simulink model "pendulum_noratiobias"  (R2020b)
settings: Solver=ode15s  StartTime=0.0  StopTime=10.0  MaxStep=0.01  RelTol=1e-5  EnableMultiTasking=on
values from neighbouring files (symbols this model uses):
  d1 = 0.5    [simu.m]    (also in simu_J1fix.m)
  d2 = 0.5    [simu.m]    (also in simu_J1fix.m)
  is_tm1 = 1    [simu.m]    (also in simu_J1fix.m)
  is_tm2 = 1    [simu.m]    (also in simu_J1fix.m)
  Izz2 = 2    [simu.m]    (also in simu_J1fix.m)
  J1 = 1    [simu.m]    (also in simu_J1fix.m)
  J2 = 1    [simu.m]    (also in simu_J1fix.m = 0.8)
  k1 = 100    [simu.m]    (also in simu_J1fix.m)
  k2 = 100    [simu.m]    (also in simu_J1fix.m = 80)
  L1 = 0.4    [simu.m]    (also in simu_J1fix.m)
  L2 = 0.2    [simu.m]    (also in simu_J1fix.m)
  Lc2 = L2/2    (= 0.1)    [simu.m]    (also in simu_J1fix.m)
  lf1 = 1    [simu.m]    (also in simu_J1fix.m = 0.1)
  m2 = 1    [simu.m]    (also in simu_J1fix.m)
undefined symbols (not defined in the file or in its folder): X, Y, Z
libraries: nesl_utility x21, sm_lib x20, fl_lib x6
settings Model: Creator=BearHsia  LastModifiedBy=BearHsia
settings DataIOCC: LimitDataPoints=on  MaxDataPoints=10000
settings OptimizationCC: LifeSpan=inf
settings DebuggingCC: AllowSymbolicDim=off  SFUnexpectedBacktrackingDiag=warning  SFNoUnconditionalDefaultTransitionDiag=warning  SFExecutionAtInitializationDiag=none  ArithmeticOperatorsInVariantConditions=warning
settings SFSimCC: SimUseLocalCustomCode=off  CustomCodeUndefinedFunction=UseInterfaceOnly
settings RTWCC: RTWUseLocalCustomCode=off
settings CodeAppCC: StateflowObjectComments=on
settings GRTTargetCC: TargetLangStandard=C89/C90 (ANSI)
settings ConfigComp: CovMetricSettings=dw  CovSaveCumulativeToWorkspaceVar=on  CovSaveSingleToWorkspaceVar=on  CovExternalEMLEnable=off  CovSFcnEnable=off
settings SimscapeCC: SimscapeLogType=all  SimscapeLogSimulationStatistics=on  SimscapeLogDataHistory=10000

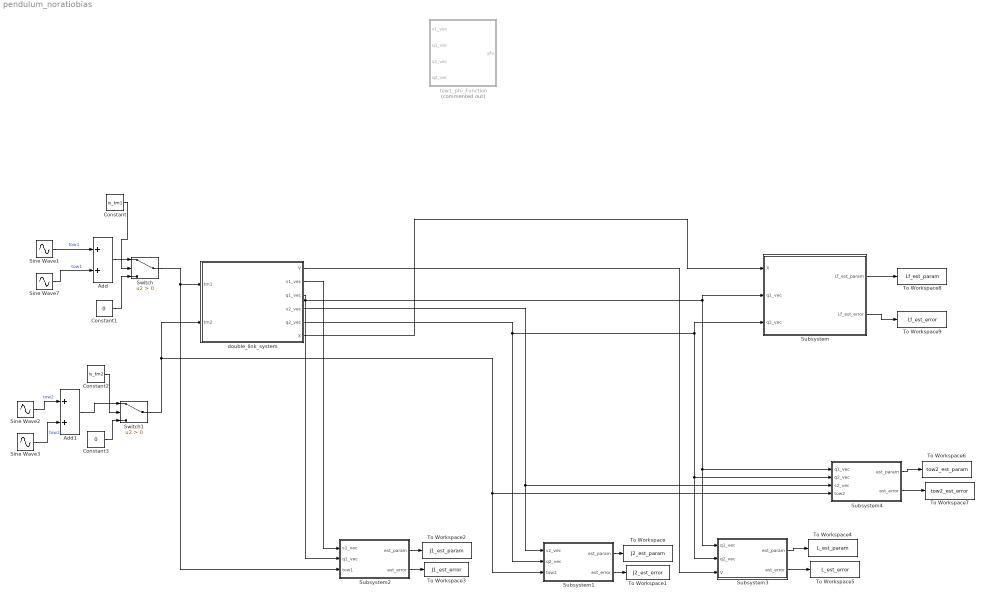
== system pendulum_noratiobias ==
  Add : Sum
  Add1 : Sum
  Constant : Constant  Value=is_tm1
  Constant1 : Constant  Value=0
  Constant2 : Constant  Value=is_tm2
  Constant3 : Constant  Value=0
  Sine Wave1 : Sin  Amplitude=2  SampleTime=0
  Sine Wave2 : Sin  Amplitude=2  SampleTime=0
  Sine Wave3 : Sin  Frequency=0.5  SampleTime=0
  Sine Wave7 : Sin  Frequency=0.5  SampleTime=0
  Subsystem : Subsystem
  Subsystem1 : Subsystem
  Subsystem2 : Subsystem
  Subsystem3 : Subsystem
  Subsystem4 : Subsystem
  Switch : Switch  Criteria=u2 > Threshold
  Switch1 : Switch  Criteria=u2 > Threshold
  To Workspace : ToWorkspace  VariableName=J2_est_param  SaveFormat=Timeseries  SampleTime=-1
  To Workspace1 : ToWorkspace  VariableName=J2_est_error  SaveFormat=Timeseries  SampleTime=-1
  To Workspace2 : ToWorkspace  VariableName=J1_est_param  SaveFormat=Timeseries  SampleTime=-1
  To Workspace3 : ToWorkspace  VariableName=J1_est_error  SaveFormat=Timeseries  SampleTime=-1
  To Workspace4 : ToWorkspace  VariableName=L_est_param  SaveFormat=Timeseries  SampleTime=-1
  To Workspace5 : ToWorkspace  VariableName=L_est_error  SaveFormat=Timeseries  SampleTime=-1
  To Workspace6 : ToWorkspace  VariableName=tow2_est_param  SaveFormat=Timeseries  SampleTime=-1
  To Workspace7 : ToWorkspace  VariableName=tow2_est_error  SaveFormat=Timeseries  SampleTime=-1
  To Workspace8 : ToWorkspace  VariableName=Lf_est_param  SaveFormat=Timeseries  SampleTime=-1
  To Workspace9 : ToWorkspace  VariableName=Lf_est_error  SaveFormat=Timeseries  SampleTime=-1
  double_link_system : Subsystem
  tow1_phi_Function : MATLAB Function  Commented=on  TreatAsAtomicUnit=on
  wires:
  double_link_system/2(s1_vec) -> Subsystem2/1(s1_vec)
  double_link_system/3(q1_vec) -> Subsystem/2(q1_vec), Subsystem4/1(q1_vec), Subsystem3/1(q1_vec), Subsystem2/2(q1_vec)
  Add/1 -> Switch/1
  Sine Wave1/1 -> Add/1  "tow1"
  Sine Wave7/1 -> Add/2  "tow1"
  double_link_system/4(s2_vec) -> Subsystem4/3(s2_vec), Subsystem1/1(s2_vec)
  double_link_system/5(q2_vec) -> Subsystem/3(q2_vec), Subsystem4/2(q2_vec), Subsystem3/2(q2_vec), Subsystem1/2(q2_vec)
  Subsystem1/1(est_param) -> To Workspace/1
  Subsystem1/2(est_error) -> To Workspace1/1
  Subsystem2/2(est_error) -> To Workspace3/1
  Subsystem2/1(est_param) -> To Workspace2/1
  Switch/1 -> Subsystem2/3(tow1), double_link_system/1(tm1)
  Constant/1 -> Switch/2
  Constant1/1 -> Switch/3
  Switch1/1 -> Subsystem4/4(tow2), Subsystem1/3(tow2), double_link_system/2(tm2)
  Constant2/1 -> Switch1/2
  Add1/1 -> Switch1/1
  Constant3/1 -> Switch1/3
  Sine Wave2/1 -> Add1/1  "tow2"
  Sine Wave3/1 -> Add1/2  "tow2"
  double_link_system/1(V) -> Subsystem3/3(V)
  Subsystem3/1(est_param) -> To Workspace4/1
  Subsystem3/2(est_error) -> To Workspace5/1
  Subsystem4/2(est_error) -> To Workspace7/1
  Subsystem4/1(est_param) -> To Workspace6/1
  double_link_system/6(X) -> Subsystem/1(X)
  Subsystem/1(Lf_est_param) -> To Workspace8/1
  Subsystem/2(Lf_est_error) -> To Workspace9/1

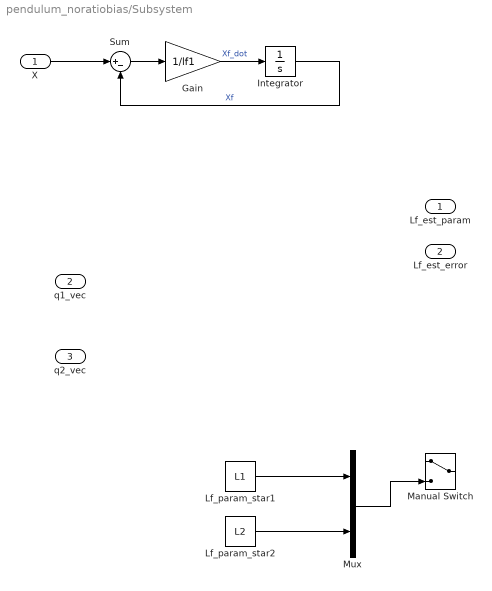
== system pendulum_noratiobias/Subsystem ==
  X : Inport
  q1_vec : Inport  Port=2
  q2_vec : Inport  Port=3
  Gain : Gain  Gain=1/lf1
  Integrator : Integrator
  Lf_param_star1 : Constant  Value=L1
  Lf_param_star2 : Constant  Value=L2
  Manual Switch : ManualSwitch
  Mux : Mux  Inputs=2
  Sum : Sum  Inputs=|+-
  Lf_est_param : Outport
  Lf_est_error : Outport  Port=2
  wires:
  Sum/1 -> Gain/1
  Gain/1 -> Integrator/1  "Xf_dot"
  X/1 -> Sum/1
  Integrator/1 -> Sum/2  "Xf"
  Mux/1 -> Manual Switch/2
  Lf_param_star1/1 -> Mux/1
  Lf_param_star2/1 -> Mux/2

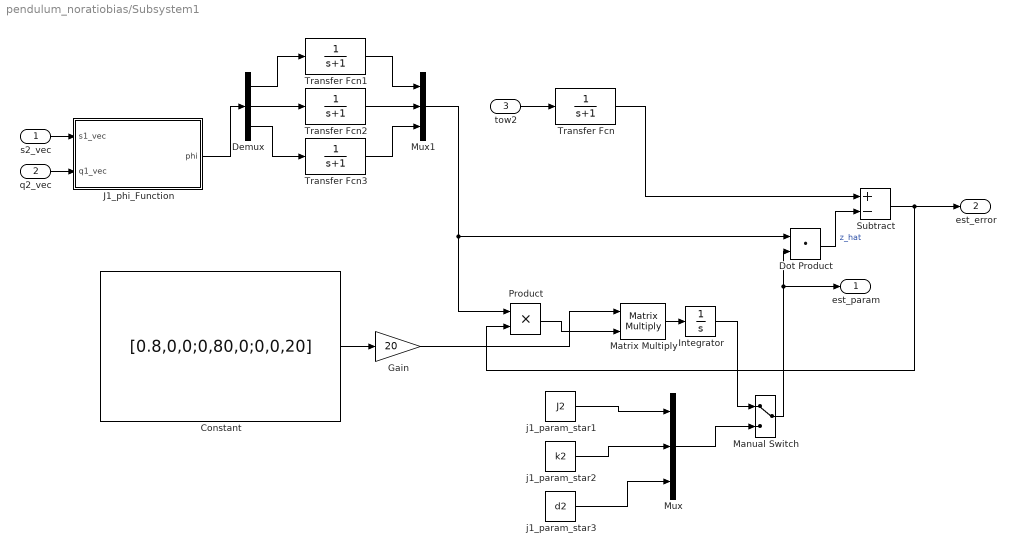
== system pendulum_noratiobias/Subsystem1 ==
  s2_vec : Inport
  q2_vec : Inport  Port=2
  tow2 : Inport  Port=3
  Constant : Constant  Value=[0.8,0,0;0,80,0;0,0,20]
  Demux : Demux  Outputs=3
  Dot Product : DotProduct  InputSameDT=on  OutDataTypeStr=Inherit: Inherit via internal rule
  Gain : Gain  Gain=20
  Integrator : Integrator  InitialCondition=[0.0001;0.0001;0.0001]
  J1_phi_Function : MATLAB Function  TreatAsAtomicUnit=on
  Manual Switch : ManualSwitch
  Matrix Multiply : Product  Multiplication=Matrix(*)
  Mux : Mux  Inputs=3
  Mux1 : Mux  Inputs=3
  Product : Product
  Subtract : Sum  Inputs=+-
  Transfer Fcn{,1..3} (4 alike) : TransferFcn  Denominator=[1 1]
  j1_param_star1 : Constant  Value=J2
  j1_param_star2 : Constant  Value=k2
  j1_param_star3 : Constant  Value=d2
  est_param : Outport
  est_error : Outport  Port=2
  wires:
  q2_vec/1 -> J1_phi_Function/2(q1_vec)
  s2_vec/1 -> J1_phi_Function/1(s1_vec)
  Integrator/1 -> Manual Switch/1
  tow2/1 -> Transfer Fcn/1
  Dot Product/1 -> Subtract/2  "z_hat"
  Matrix Multiply/1 -> Integrator/1
  Subtract/1 -> est_error/1, Product/2
  j1_param_star1/1 -> Mux/1
  j1_param_star2/1 -> Mux/2
  j1_param_star3/1 -> Mux/3
  Mux/1 -> Manual Switch/2
  Product/1 -> Matrix Multiply/2
  Gain/1 -> Matrix Multiply/1
  J1_phi_Function/1(phi) -> Demux/1
  Manual Switch/1 -> est_param/1, Dot Product/2
  Transfer Fcn/1 -> Subtract/1
  Transfer Fcn1/1 -> Mux1/1
  Transfer Fcn2/1 -> Mux1/2
  Transfer Fcn3/1 -> Mux1/3
  Demux/3 -> Transfer Fcn3/1
  Demux/2 -> Transfer Fcn2/1
  Demux/1 -> Transfer Fcn1/1
  Mux1/1 -> Product/1, Dot Product/1
  Constant/1 -> Gain/1

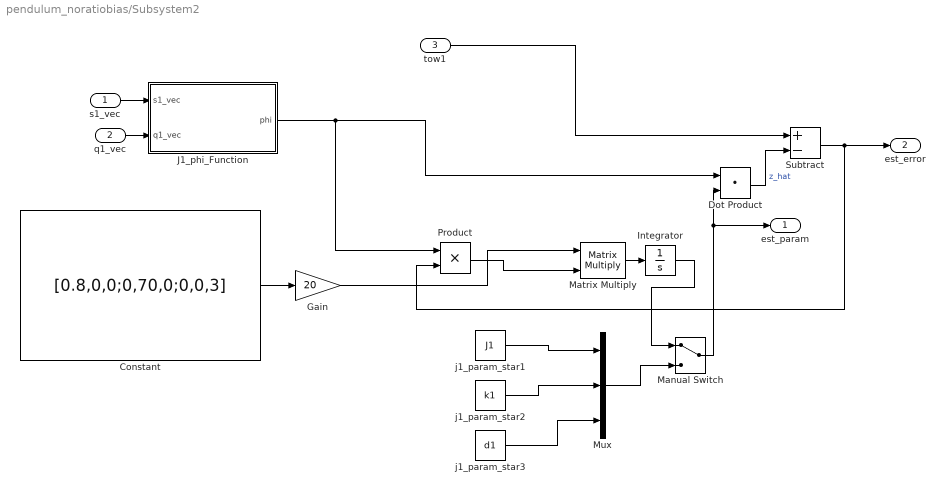
== system pendulum_noratiobias/Subsystem2 ==
  s1_vec : Inport
  q1_vec : Inport  Port=2
  tow1 : Inport  Port=3
  Constant : Constant  Value=[0.8,0,0;0,70,0;0,0,3]
  Dot Product : DotProduct  InputSameDT=on  OutDataTypeStr=Inherit: Inherit via internal rule
  Gain : Gain  Gain=20
  Integrator : Integrator  InitialCondition=[0;0;0]
  J1_phi_Function : MATLAB Function  TreatAsAtomicUnit=on
  Manual Switch : ManualSwitch
  Matrix Multiply : Product  Multiplication=Matrix(*)
  Mux : Mux  Inputs=3
  Product : Product
  Subtract : Sum  Inputs=+-
  j1_param_star1 : Constant  Value=J1
  j1_param_star2 : Constant  Value=k1
  j1_param_star3 : Constant  Value=d1
  est_param : Outport
  est_error : Outport  Port=2
  wires:
  q1_vec/1 -> J1_phi_Function/2(q1_vec)
  s1_vec/1 -> J1_phi_Function/1(s1_vec)
  Integrator/1 -> Manual Switch/1
  tow1/1 -> Subtract/1
  Dot Product/1 -> Subtract/2  "z_hat"
  Matrix Multiply/1 -> Integrator/1
  Subtract/1 -> est_error/1, Product/2
  j1_param_star1/1 -> Mux/1
  j1_param_star2/1 -> Mux/2
  j1_param_star3/1 -> Mux/3
  Mux/1 -> Manual Switch/2
  Product/1 -> Matrix Multiply/2
  Constant/1 -> Gain/1
  Gain/1 -> Matrix Multiply/1
  J1_phi_Function/1(phi) -> Dot Product/1, Product/1
  Manual Switch/1 -> est_param/1, Dot Product/2

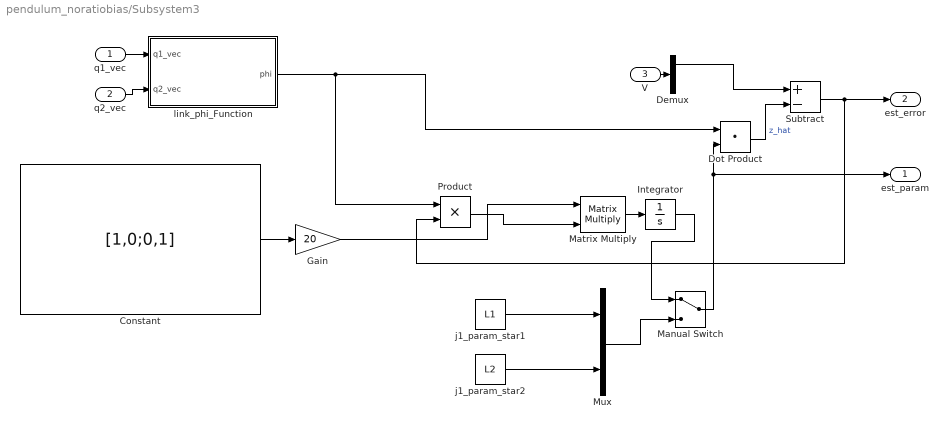
== system pendulum_noratiobias/Subsystem3 ==
  q1_vec : Inport
  q2_vec : Inport  Port=2
  V : Inport  Port=3
  Constant : Constant  Value=[1,0;0,1]
  Demux : Demux  Outputs=2
  Dot Product : DotProduct  InputSameDT=on  OutDataTypeStr=Inherit: Inherit via internal rule
  Gain : Gain  Gain=20
  Integrator : Integrator  InitialCondition=[0;0]
  Manual Switch : ManualSwitch
  Matrix Multiply : Product  Multiplication=Matrix(*)
  Mux : Mux  Inputs=2
  Product : Product
  Subtract : Sum  Inputs=+-
  j1_param_star1 : Constant  Value=L1
  j1_param_star2 : Constant  Value=L2
  link_phi_Function : MATLAB Function  TreatAsAtomicUnit=on
  est_param : Outport
  est_error : Outport  Port=2
  wires:
  Integrator/1 -> Manual Switch/1
  Dot Product/1 -> Subtract/2  "z_hat"
  Matrix Multiply/1 -> Integrator/1
  Subtract/1 -> est_error/1, Product/2
  j1_param_star1/1 -> Mux/1
  j1_param_star2/1 -> Mux/2
  Mux/1 -> Manual Switch/2
  Product/1 -> Matrix Multiply/2
  Constant/1 -> Gain/1
  Gain/1 -> Matrix Multiply/1
  link_phi_Function/1(phi) -> Dot Product/1, Product/1
  Manual Switch/1 -> est_param/1, Dot Product/2
  q2_vec/1 -> link_phi_Function/2(q2_vec)
  q1_vec/1 -> link_phi_Function/1(q1_vec)
  V/1 -> Demux/1
  Demux/1 -> Subtract/1

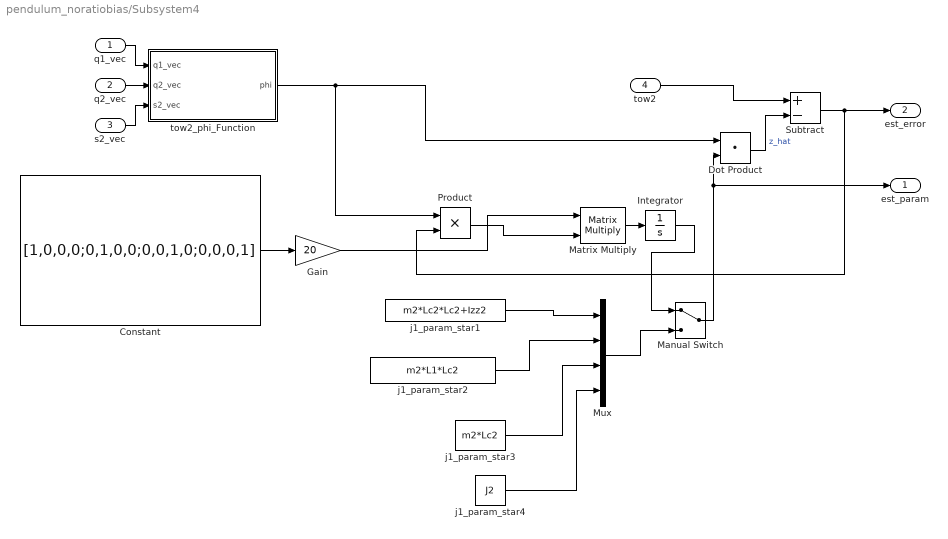
== system pendulum_noratiobias/Subsystem4 ==
  q1_vec : Inport
  q2_vec : Inport  Port=2
  s2_vec : Inport  Port=3
  tow2 : Inport  Port=4
  Constant : Constant  Value=[1,0,0,0;0,1,0,0;0,0,1,0;0,0,0,1]
  Dot Product : DotProduct  InputSameDT=on  OutDataTypeStr=Inherit: Inherit via internal rule
  Gain : Gain  Gain=20
  Integrator : Integrator  InitialCondition=[0;0;0;0]
  Manual Switch : ManualSwitch
  Matrix Multiply : Product  Multiplication=Matrix(*)
  Mux : Mux
  Product : Product
  Subtract : Sum  Inputs=+-
  j1_param_star1 : Constant  Value=m2*Lc2*Lc2+Izz2
  j1_param_star2 : Constant  Value=m2*L1*Lc2
  j1_param_star3 : Constant  Value=m2*Lc2
  j1_param_star4 : Constant  Value=J2
  tow2_phi_Function : MATLAB Function  TreatAsAtomicUnit=on
  est_param : Outport
  est_error : Outport  Port=2
  wires:
  Integrator/1 -> Manual Switch/1
  Dot Product/1 -> Subtract/2  "z_hat"
  Matrix Multiply/1 -> Integrator/1
  Subtract/1 -> est_error/1, Product/2
  j1_param_star1/1 -> Mux/1
  j1_param_star2/1 -> Mux/2
  Mux/1 -> Manual Switch/2
  Product/1 -> Matrix Multiply/2
  Constant/1 -> Gain/1
  Gain/1 -> Matrix Multiply/1
  tow2_phi_Function/1(phi) -> Dot Product/1, Product/1
  Manual Switch/1 -> est_param/1, Dot Product/2
  q2_vec/1 -> tow2_phi_Function/2(q2_vec)
  q1_vec/1 -> tow2_phi_Function/1(q1_vec)
  tow2/1 -> Subtract/1
  s2_vec/1 -> tow2_phi_Function/3(s2_vec)
  j1_param_star3/1 -> Mux/3
  j1_param_star4/1 -> Mux/4

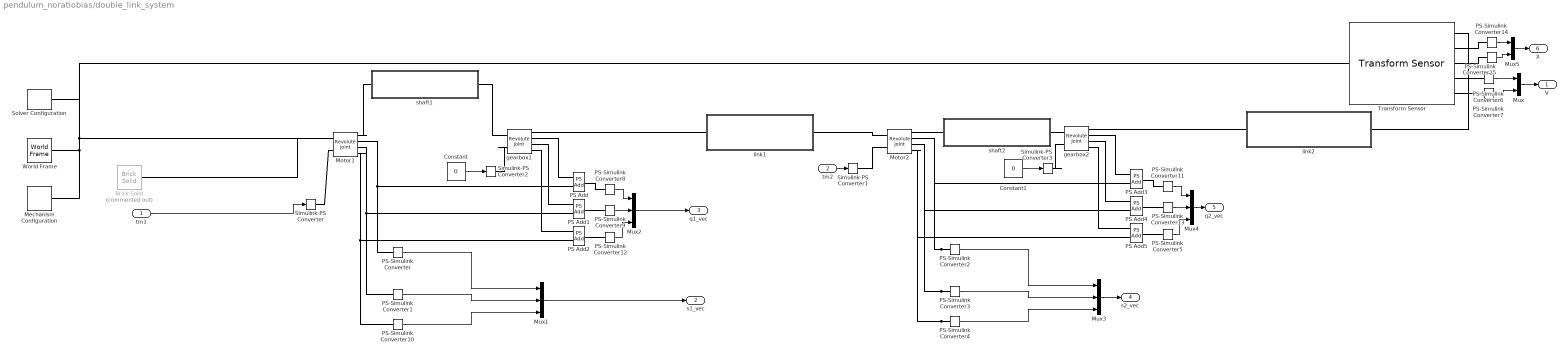
== system pendulum_noratiobias/double_link_system ==
  tm1 : Inport
  tm2 : Inport  Port=2
  Brick Solid : sm_lib/Body Elements/Brick Solid  Commented=on  GraphicAmbientColor=[0.15 0.15 0.15 1.0]  BasedOnType=Density  BrickDimensions=[4 4 4]  BrickDimensionUnits=cm  CenterOfMass=[0 0 0]  CenterOfMassUnits=m  GraphicDiffuseColor=[0.8 0.45 0]  Density=1000  DensityUnits=kg/m^3  DoExposeReferenceFrame=on  GraphicEmissiveColor=[0.0 0.0 0.0 1.0]  ExportEntireGeometry=off  SerializedFrames=<Frames/>  MarkerShape=Sphere  MarkerSize=10  GraphicType=FromGeometry  InertiaType=CalculateFromGeometry  Mass=1  MassUnits=kg  MomentsOfInertia=[1 1 1]  MomentsOfInertiaUnits=kg*m^2  GraphicOpacity=1.0  ProductsOfInertia=[0 0 0]  ProductsOfInertiaUnits=kg*m^2  GraphicShininess=75  GraphicSpecularColor=[0.5 0.5 0.5 1.0]  GraphicVisPropType=SimpleVisualProperties
  Constant : Constant  Value=0
  Constant1 : Constant  Value=0
  Mechanism Configuration : sm_lib/Utilities/Mechanism Configuration  UniformGravity=Constant  GravityVector=[0 -9.81 0]  GravityVectorUnits=m/s^2  GravityUnits=m/s^2  LinearizationDelta=0.001  JointModeTransitionNonlinearIterations=2
  Motor1 : sm_lib/Joints/Revolute Joint  JointMode=Normal  SenseConstraintForce=off  SenseConstraintForceX=off  SenseConstraintForceY=off  SenseConstraintForceZ=off  SenseConstraintTorque=off  SenseConstraintTorqueX=off  SenseConstraintTorqueY=off  SenseConstraintTorqueZ=off  SenseTotalForce=off  SenseTotalForceX=off  SenseTotalForceY=off  SenseTotalForceZ=off  SenseTotalTorque=off  SenseTotalTorqueX=off  SenseTotalTorqueY=off  SenseTotalTorqueZ=off  CompositeWrenchDir=FollowerOnBase  CompositeWrenchFrame=BaseFrame  EquilibriumPosition=-pi/2  EquilibriumPositionUnits=rad  SpringStiffness=0  SpringStiffnessUnits=N*m/rad  DampingCoefficient=0  DampingCoefficientUnits=N*m/(rad/s)  TorqueActuationMode=InputTorque  MotionActuationMode=ComputedMotion  SensePosition=on  SenseVelocity=on  SenseAcceleration=on  SenseTorqueForce=off  SenseLowerLimitTorqueForce=off  SenseUpperLimitTorqueForce=off  LowerLimitSpecify=off  LowerLimitBound=-90  LowerLimitBoundUnits=deg  LowerLimitStiffness=1e4  LowerLimitStiffnessUnits=N*m/deg  LowerLimitDamping=10  LowerLimitDampingUnits=N*m/(deg/s)  LowerLimitTransitionRegionWidth=0.1  LowerLimitTransitionRegionWidthUnits=deg  UpperLimitSpecify=off  UpperLimitBound=90  UpperLimitBoundUnits=deg  UpperLimitStiffness=1e4  UpperLimitStiffnessUnits=N*m/deg  UpperLimitDamping=10  UpperLimitDampingUnits=N*m/(deg/s)  UpperLimitTransitionRegionWidth=0.1  UpperLimitTransitionRegionWidthUnits=deg  PositionTargetSpecify=on  PositionTargetPriority=High  PositionTargetValue=-pi/2  PositionTargetValueUnits=rad  VelocityTargetSpecify=off  VelocityTargetPriority=High  VelocityTargetValue=0  VelocityTargetValueUnits=deg/s
  Motor2 : sm_lib/Joints/Revolute Joint  JointMode=Normal  SenseConstraintForce=off  SenseConstraintForceX=off  SenseConstraintForceY=off  SenseConstraintForceZ=off  SenseConstraintTorque=off  SenseConstraintTorqueX=off  SenseConstraintTorqueY=off  SenseConstraintTorqueZ=off  SenseTotalForce=off  SenseTotalForceX=off  SenseTotalForceY=off  SenseTotalForceZ=off  SenseTotalTorque=off  SenseTotalTorqueX=off  SenseTotalTorqueY=off  SenseTotalTorqueZ=off  CompositeWrenchDir=FollowerOnBase  CompositeWrenchFrame=BaseFrame  EquilibriumPosition=0  EquilibriumPositionUnits=rad  SpringStiffness=0  SpringStiffnessUnits=N*m/rad  DampingCoefficient=0  DampingCoefficientUnits=N*m/(rad/s)  TorqueActuationMode=InputTorque  MotionActuationMode=ComputedMotion  SensePosition=on  SenseVelocity=on  SenseAcceleration=on  SenseTorqueForce=off  SenseLowerLimitTorqueForce=off  SenseUpperLimitTorqueForce=off  LowerLimitSpecify=off  LowerLimitBound=-90  LowerLimitBoundUnits=deg  LowerLimitStiffness=1e4  LowerLimitStiffnessUnits=N*m/deg  LowerLimitDamping=10  LowerLimitDampingUnits=N*m/(deg/s)  LowerLimitTransitionRegionWidth=0.1  LowerLimitTransitionRegionWidthUnits=deg  UpperLimitSpecify=off  UpperLimitBound=90  UpperLimitBoundUnits=deg  UpperLimitStiffness=1e4  UpperLimitStiffnessUnits=N*m/deg  UpperLimitDamping=10  UpperLimitDampingUnits=N*m/(deg/s)  UpperLimitTransitionRegionWidth=0.1  UpperLimitTransitionRegionWidthUnits=deg  PositionTargetSpecify=on  PositionTargetPriority=High  PositionTargetValue=0  PositionTargetValueUnits=rad  VelocityTargetSpecify=off  VelocityTargetPriority=High  VelocityTargetValue=0  VelocityTargetValueUnits=deg/s
  Mux : Mux  Inputs=2
  Mux{1..4} (4 alike) : Mux  Inputs=3
  Mux5 : Mux  Inputs=2
  PS Add{,1..5} (6 alike) : fl_lib/Physical Signals/Functions/PS Add
  PS-Simulink Converter{,1..15} (16 alike) : nesl_utility/PS-Simulink Converter  PhysicalDomain=network_engine_domain  SubClassName=ps_output  LeftPortType=input  RightPortType=output  PseudoPeriodic=off  Frequencies=[]  Unit=inherit  AffineConversion=off
  Simulink-PS Converter{,1..3} (4 alike) : nesl_utility/Simulink-PS Converter  PhysicalDomain=network_engine_domain  SubClassName=ps_input  LeftPortType=input  RightPortType=output  PseudoPeriodic=off  Frequencies=[]  NoiseDistribution=none  NoiseParameters=[]  Unit=1  AffineConversion=off  FilteringAndDerivatives=provide  SimscapeFilterOrder=1  InputFilterTimeConstant=0.001  UdotUserProvided=0
  Solver Configuration : nesl_utility/Solver Configuration  PhysicalDomain=network_engine_domain  SubClassName=solver  LeftPortType=input  RightPortType=generic  Tones=[]  Harmonics=[]  SimulateNoise=off  Profile=off  UseLocalSampling=off  EnableSwitchedLinearOptims=on  FrequencyDomain=off  UseCCode=off  RelTol=0.001  AbsTol=1e-06  MinStep=1e-09  ToWorkspace=off  RevertToSquareIcSolve=off  NumHomotopyIterations=100  PhasorMode=off  PhasorModeNumHarmonics=1  DoDC=on  ResidualTolerance=1e-09  UseLocalSolver=off  LocalSolverChoice=NE_BACKWARD_EULER_ADVANCER  LocalSolverSampleTime=0.001  DoFixedCost=off  MaxNonlinIter=3  MaxModeIter=2  ComputeImpulses=off  ImpulseIterations=2  LinearAlgebra=Sparse  EquationFormulation=NE_TIME_EF  DelaysMemoryBudget=1024  AutomaticFiltering=on  FilteringTimeConstant=0.001  PartitionStorageMethod=AS_NEEDED  PartitionMemoryBudget=1024  PartitionMethod=FAST
  Transform Sensor : sm_lib/Frames and Transforms/Transform Sensor  MeasurementFrame=World  SenseAngle=off  SenseAxis=off  SenseAngle1=off  SenseAngle2=off  SenseAngle3=off  SenseQ=off  SenseR=off  SenseOmegaX=off  SenseOmegaY=off  SenseOmegaZ=off  SenseOmega1=off  SenseOmega2=off  SenseOmega3=off  SenseQDot=off  SenseRDot=off  SenseAlphaX=off  SenseAlphaY=off  SenseAlphaZ=off  SenseAlpha1=off  SenseAlpha2=off  SenseAlpha3=off  SenseQDDot=off  SenseRDDot=off  SenseX=on  SenseY=on  SenseZ=off  SenseRad=off  SenseAzim=off  SenseDist=off  SenseInc=off  SenseXDot=on  SenseYDot=on  SenseZDot=off  SenseRadDot=off  SenseAzimDot=off  SenseDistDot=off  SenseIncDot=off  SenseXDDot=off  SenseYDDot=off  SenseZDDot=off  SenseRadDDot=off  SenseAzimDDot=off  SenseDistDDot=off  SenseIncDDot=off
  World Frame : sm_lib/Frames and Transforms/World Frame
  gearbox1 : sm_lib/Joints/Revolute Joint  JointMode=Normal  SenseConstraintForce=off  SenseConstraintForceX=off  SenseConstraintForceY=off  SenseConstraintForceZ=off  SenseConstraintTorque=off  SenseConstraintTorqueX=off  SenseConstraintTorqueY=off  SenseConstraintTorqueZ=off  SenseTotalForce=off  SenseTotalForceX=off  SenseTotalForceY=off  SenseTotalForceZ=off  SenseTotalTorque=off  SenseTotalTorqueX=off  SenseTotalTorqueY=off  SenseTotalTorqueZ=off  CompositeWrenchDir=FollowerOnBase  CompositeWrenchFrame=BaseFrame  EquilibriumPosition=0  EquilibriumPositionUnits=rad  SpringStiffness=k1  SpringStiffnessUnits=N*m/rad  DampingCoefficient=d1  DampingCoefficientUnits=N*m/(rad/s)  TorqueActuationMode=InputTorque  MotionActuationMode=ComputedMotion  SensePosition=on  SenseVelocity=on  SenseAcceleration=on  SenseTorqueForce=off  SenseLowerLimitTorqueForce=off  SenseUpperLimitTorqueForce=off  LowerLimitSpecify=off  LowerLimitBound=-90  LowerLimitBoundUnits=deg  LowerLimitStiffness=1e4  LowerLimitStiffnessUnits=N*m/deg  LowerLimitDamping=10  LowerLimitDampingUnits=N*m/(deg/s)  LowerLimitTransitionRegionWidth=0.1  LowerLimitTransitionRegionWidthUnits=deg  UpperLimitSpecify=off  UpperLimitBound=90  UpperLimitBoundUnits=deg  UpperLimitStiffness=1e4  UpperLimitStiffnessUnits=N*m/deg  UpperLimitDamping=10  UpperLimitDampingUnits=N*m/(deg/s)  UpperLimitTransitionRegionWidth=0.1  UpperLimitTransitionRegionWidthUnits=deg  PositionTargetSpecify=on  PositionTargetPriority=High  PositionTargetValue=0  PositionTargetValueUnits=rad  VelocityTargetSpecify=off  VelocityTargetPriority=High  VelocityTargetValue=0  VelocityTargetValueUnits=deg/s
  gearbox2 : sm_lib/Joints/Revolute Joint  JointMode=Normal  SenseConstraintForce=off  SenseConstraintForceX=off  SenseConstraintForceY=off  SenseConstraintForceZ=off  SenseConstraintTorque=off  SenseConstraintTorqueX=off  SenseConstraintTorqueY=off  SenseConstraintTorqueZ=off  SenseTotalForce=off  SenseTotalForceX=off  SenseTotalForceY=off  SenseTotalForceZ=off  SenseTotalTorque=off  SenseTotalTorqueX=off  SenseTotalTorqueY=off  SenseTotalTorqueZ=off  CompositeWrenchDir=FollowerOnBase  CompositeWrenchFrame=BaseFrame  EquilibriumPosition=0  EquilibriumPositionUnits=rad  SpringStiffness=k2  SpringStiffnessUnits=N*m/rad  DampingCoefficient=d2  DampingCoefficientUnits=N*m/(rad/s)  TorqueActuationMode=InputTorque  MotionActuationMode=ComputedMotion  SensePosition=on  SenseVelocity=on  SenseAcceleration=on  SenseTorqueForce=off  SenseLowerLimitTorqueForce=off  SenseUpperLimitTorqueForce=off  LowerLimitSpecify=off  LowerLimitBound=-90  LowerLimitBoundUnits=deg  LowerLimitStiffness=1e4  LowerLimitStiffnessUnits=N*m/deg  LowerLimitDamping=10  LowerLimitDampingUnits=N*m/(deg/s)  LowerLimitTransitionRegionWidth=0.1  LowerLimitTransitionRegionWidthUnits=deg  UpperLimitSpecify=off  UpperLimitBound=90  UpperLimitBoundUnits=deg  UpperLimitStiffness=1e4  UpperLimitStiffnessUnits=N*m/deg  UpperLimitDamping=10  UpperLimitDampingUnits=N*m/(deg/s)  UpperLimitTransitionRegionWidth=0.1  UpperLimitTransitionRegionWidthUnits=deg  PositionTargetSpecify=on  PositionTargetPriority=High  PositionTargetValue=0  PositionTargetValueUnits=rad  VelocityTargetSpecify=off  VelocityTargetPriority=High  VelocityTargetValue=0  VelocityTargetValueUnits=deg/s
  link1 : Subsystem  mask{rgb=[0.25 0.4 0.7], Ixx=1, Iyy=1, Izz=3, M=1, L=L1, W=0.04, H=0.04}
      mask prompts: rgb "Color [R G B]"
  link2 : Subsystem  mask{rgb=[0.25 0.4 0.7], Ixx=1, Iyy=1, Izz=Izz2, M=m2, L=L2, W=0.04, H=0.04}
      mask prompts: rgb "Color [R G B]"
  shaft1 : Subsystem  mask{rgb=[0 1 0], Ixx=0, Iyy=0, Izz=J1, M=0.1, L=0.2, W=0.004, H=0.004}
      mask prompts: rgb "Color [R G B]"
  shaft2 : Subsystem  mask{rgb=[0 1 0], Ixx=0, Iyy=0, Izz=J2, M=0.1, L=0.2, W=0.004, H=0.004}
      mask prompts: rgb "Color [R G B]"
  V : Outport
  s1_vec : Outport  Port=2
  q1_vec : Outport  Port=3
  s2_vec : Outport  Port=4
  q2_vec : Outport  Port=5
  X : Outport  Port=6
  wires:
  tm2/1 -> Simulink-PS Converter1/1
  tm1/1 -> Simulink-PS Converter/1
  PS-Simulink Converter6/1 -> Mux/1
  PS-Simulink Converter7/1 -> Mux/2
  Mux/1 -> V/1
  PS-Simulink Converter9/1 -> Mux2/2
  PS-Simulink Converter8/1 -> Mux2/1
  PS-Simulink Converter12/1 -> Mux2/3
  Mux1/1 -> s1_vec/1
  Mux2/1 -> q1_vec/1
  PS-Simulink Converter/1 -> Mux1/1
  PS-Simulink Converter1/1 -> Mux1/2
  PS-Simulink Converter10/1 -> Mux1/3
  Mux3/1 -> s2_vec/1
  PS-Simulink Converter2/1 -> Mux3/1
  PS-Simulink Converter4/1 -> Mux3/3
  PS-Simulink Converter5/1 -> Mux4/3
  PS-Simulink Converter11/1 -> Mux4/1
  Mux4/1 -> q2_vec/1
  PS-Simulink Converter13/1 -> Mux4/2
  PS-Simulink Converter3/1 -> Mux3/2
  Constant/1 -> Simulink-PS Converter2/1
  Constant1/1 -> Simulink-PS Converter3/1
  Mux5/1 -> X/1
  PS-Simulink Converter14/1 -> Mux5/1
  PS-Simulink Converter15/1 -> Mux5/2
  connections:
  Simulink-PS Converter/RConn1 -- Motor1/LConn2
  World Frame/RConn1 -- Mechanism Configuration/RConn1 -- Transform Sensor/LConn1 -- Solver Configuration/RConn1 -- Brick Solid/RConn1 -- Motor1/LConn1
  Motor1/RConn4 -- PS Add2/LConn2 -- PS-Simulink Converter10/LConn1
  Motor1/RConn2 -- PS Add/LConn2 -- PS-Simulink Converter/LConn1
  link2/RConn1 -- Transform Sensor/RConn1
  Transform Sensor/RConn5 -- PS-Simulink Converter7/LConn1
  gearbox1/RConn3 -- PS Add1/LConn1
  PS Add1/RConn1 -- PS-Simulink Converter9/LConn1
  gearbox1/RConn4 -- PS Add2/LConn1
  PS Add/RConn1 -- PS-Simulink Converter8/LConn1
  Motor1/RConn3 -- PS Add1/LConn2 -- PS-Simulink Converter1/LConn1
  Transform Sensor/RConn4 -- PS-Simulink Converter6/LConn1
  gearbox1/RConn2 -- PS Add/LConn1
  PS-Simulink Converter12/LConn1 -- PS Add2/RConn1
  PS-Simulink Converter4/LConn1 -- Motor2/RConn4 -- PS Add5/LConn2
  PS-Simulink Converter3/LConn1 -- Motor2/RConn3 -- PS Add4/LConn2
  PS-Simulink Converter2/LConn1 -- Motor2/RConn2 -- PS Add3/LConn2
  gearbox2/RConn1 -- link2/LConn1
  gearbox2/RConn2 -- PS Add3/LConn1
  shaft2/LConn1 -- Motor2/RConn1
  gearbox2/RConn3 -- PS Add4/LConn1
  PS-Simulink Converter5/LConn1 -- PS Add5/RConn1
  PS Add3/RConn1 -- PS-Simulink Converter11/LConn1
  shaft2/RConn1 -- gearbox2/LConn1
  gearbox2/RConn4 -- PS Add5/LConn1
  PS Add4/RConn1 -- PS-Simulink Converter13/LConn1
  link1/RConn1 -- Motor2/LConn1
  Simulink-PS Converter1/RConn1 -- Motor2/LConn2
  gearbox1/LConn2 -- Simulink-PS Converter2/RConn1
  Simulink-PS Converter3/RConn1 -- gearbox2/LConn2
  Motor1/RConn1 -- shaft1/LConn1
  shaft1/RConn1 -- gearbox1/LConn1
  gearbox1/RConn1 -- link1/LConn1
  Transform Sensor/RConn2 -- PS-Simulink Converter14/LConn1
  Transform Sensor/RConn3 -- PS-Simulink Converter15/LConn1

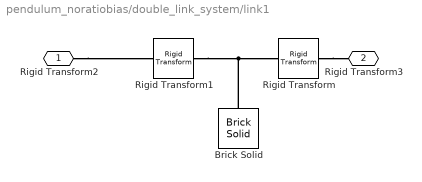
== system pendulum_noratiobias/double_link_system/link1 ==
  Brick Solid : sm_lib/Body Elements/Brick Solid  GraphicAmbientColor=[0.15 0.15 0.15 1.0]  BasedOnType=Density  BrickDimensions=[L W H]  BrickDimensionUnits=m  CenterOfMass=[0 0 0]  CenterOfMassUnits=m  GraphicDiffuseColor=rgb  Density=2700  DensityUnits=kg/m^3  DoExposeReferenceFrame=on  GraphicEmissiveColor=[0.0 0.0 0.0 1.0]  ExportEntireGeometry=off  SerializedFrames=<Frames/>  MarkerShape=Sphere  MarkerSize=10  GraphicType=FromGeometry  InertiaType=Custom  Mass=M  MassUnits=kg  MomentsOfInertia=[Ixx Iyy Izz]  MomentsOfInertiaUnits=kg*m^2  GraphicOpacity=1.0  ProductsOfInertia=[0 0 0]  ProductsOfInertiaUnits=kg*m^2  GraphicShininess=75  GraphicSpecularColor=[0.5 0.5 0.5 1.0]  GraphicVisPropType=SimpleVisualProperties
  Rigid Transform : sm_lib/Frames and Transforms/Rigid Transform  TranslationMethod=StandardAxis  TranslationStandardOffset=L/2  TranslationLengthUnit=m  TranslationStandardAxis=+X  TranslationCartesianOffset=[0 0 0]  TranslationROffset=0  TranslationROffsetUnits=m  TranslationZOffset=0  TranslationZOffsetUnits=m  TranslationThetaOffset=0  TranslationThetaOffsetUnits=deg  RotationMethod=None  RotationAngleUnits=deg  RotationStandardAxis=+Z  RotationAngle=0.0  RotationArbitraryAxis=[0 0 1]  FollAlignAxisA=+X  BaseAlignAxisA=+Y  FollAlignAxisB=+Y  BaseAlignAxisB=+Z  RotationSequenceAxes=FollowerAxes  RotationSequence=XYX  RotationSequenceAngles=[0 0 0]  RotationSequenceAnglesUnits=deg  RotationMatrix=[1 0 0; 0 1 0; 0 0 1]
  Rigid Transform1 : sm_lib/Frames and Transforms/Rigid Transform  TranslationMethod=StandardAxis  TranslationStandardOffset=L/2  TranslationLengthUnit=m  TranslationStandardAxis=-X  TranslationCartesianOffset=[0 0 0]  TranslationROffset=0  TranslationROffsetUnits=m  TranslationZOffset=0  TranslationZOffsetUnits=m  TranslationThetaOffset=0  TranslationThetaOffsetUnits=deg  RotationMethod=None  RotationAngleUnits=deg  RotationStandardAxis=-X  RotationAngle=0.0  RotationArbitraryAxis=[0 0 1]  FollAlignAxisA=+X  BaseAlignAxisA=+Y  FollAlignAxisB=+Y  BaseAlignAxisB=+Z  RotationSequenceAxes=FollowerAxes  RotationSequence=XYX  RotationSequenceAngles=[0 0 0]  RotationSequenceAnglesUnits=deg  RotationMatrix=[1 0 0; 0 1 0; 0 0 1]
  Rigid Transform2 : PMIOPort  Side=Left
  Rigid Transform3 : PMIOPort  Port=2  Side=Right
  connections:
  Rigid Transform1/LConn1 -- Rigid Transform/LConn1 -- Brick Solid/RConn1
  Rigid Transform/RConn1 -- Rigid Transform3/RConn1
  Rigid Transform2/RConn1 -- Rigid Transform1/RConn1

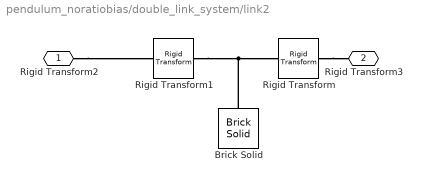
== system pendulum_noratiobias/double_link_system/link2 ==
  Brick Solid : sm_lib/Body Elements/Brick Solid  GraphicAmbientColor=[0.15 0.15 0.15 1.0]  BasedOnType=Density  BrickDimensions=[L W H]  BrickDimensionUnits=m  CenterOfMass=[0 0 0]  CenterOfMassUnits=m  GraphicDiffuseColor=rgb  Density=2700  DensityUnits=kg/m^3  DoExposeReferenceFrame=on  GraphicEmissiveColor=[0.0 0.0 0.0 1.0]  ExportEntireGeometry=off  SerializedFrames=<Frames/>  MarkerShape=Sphere  MarkerSize=10  GraphicType=FromGeometry  InertiaType=Custom  Mass=M  MassUnits=kg  MomentsOfInertia=[Ixx Iyy Izz]  MomentsOfInertiaUnits=kg*m^2  GraphicOpacity=1.0  ProductsOfInertia=[0 0 0]  ProductsOfInertiaUnits=kg*m^2  GraphicShininess=75  GraphicSpecularColor=[0.5 0.5 0.5 1.0]  GraphicVisPropType=SimpleVisualProperties
  Rigid Transform : sm_lib/Frames and Transforms/Rigid Transform  TranslationMethod=StandardAxis  TranslationStandardOffset=L/2  TranslationLengthUnit=m  TranslationStandardAxis=+X  TranslationCartesianOffset=[0 0 0]  TranslationROffset=0  TranslationROffsetUnits=m  TranslationZOffset=0  TranslationZOffsetUnits=m  TranslationThetaOffset=0  TranslationThetaOffsetUnits=deg  RotationMethod=None  RotationAngleUnits=deg  RotationStandardAxis=+Z  RotationAngle=0.0  RotationArbitraryAxis=[0 0 1]  FollAlignAxisA=+X  BaseAlignAxisA=+Y  FollAlignAxisB=+Y  BaseAlignAxisB=+Z  RotationSequenceAxes=FollowerAxes  RotationSequence=XYX  RotationSequenceAngles=[0 0 0]  RotationSequenceAnglesUnits=deg  RotationMatrix=[1 0 0; 0 1 0; 0 0 1]
  Rigid Transform1 : sm_lib/Frames and Transforms/Rigid Transform  TranslationMethod=StandardAxis  TranslationStandardOffset=L/2  TranslationLengthUnit=m  TranslationStandardAxis=-X  TranslationCartesianOffset=[0 0 0]  TranslationROffset=0  TranslationROffsetUnits=m  TranslationZOffset=0  TranslationZOffsetUnits=m  TranslationThetaOffset=0  TranslationThetaOffsetUnits=deg  RotationMethod=None  RotationAngleUnits=deg  RotationStandardAxis=-X  RotationAngle=0.0  RotationArbitraryAxis=[0 0 1]  FollAlignAxisA=+X  BaseAlignAxisA=+Y  FollAlignAxisB=+Y  BaseAlignAxisB=+Z  RotationSequenceAxes=FollowerAxes  RotationSequence=XYX  RotationSequenceAngles=[0 0 0]  RotationSequenceAnglesUnits=deg  RotationMatrix=[1 0 0; 0 1 0; 0 0 1]
  Rigid Transform2 : PMIOPort  Side=Left
  Rigid Transform3 : PMIOPort  Port=2  Side=Right
  connections:
  Rigid Transform1/LConn1 -- Rigid Transform/LConn1 -- Brick Solid/RConn1
  Rigid Transform/RConn1 -- Rigid Transform3/RConn1
  Rigid Transform2/RConn1 -- Rigid Transform1/RConn1

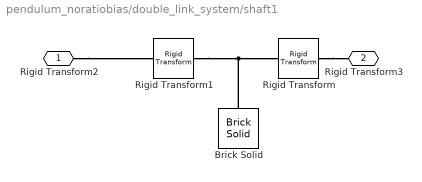
== system pendulum_noratiobias/double_link_system/shaft1 ==
  Brick Solid : sm_lib/Body Elements/Brick Solid  GraphicAmbientColor=[0.15 0.15 0.15 1.0]  BasedOnType=Density  BrickDimensions=[L W H]  BrickDimensionUnits=m  CenterOfMass=[0 0 0]  CenterOfMassUnits=m  GraphicDiffuseColor=rgb  Density=2700  DensityUnits=kg/m^3  DoExposeReferenceFrame=on  GraphicEmissiveColor=[0.0 0.0 0.0 1.0]  ExportEntireGeometry=off  SerializedFrames=<Frames/>  MarkerShape=Sphere  MarkerSize=10  GraphicType=FromGeometry  InertiaType=Custom  Mass=M  MassUnits=kg  MomentsOfInertia=[Ixx Iyy Izz]  MomentsOfInertiaUnits=kg*m^2  GraphicOpacity=1.0  ProductsOfInertia=[0 0 0]  ProductsOfInertiaUnits=kg*m^2  GraphicShininess=75  GraphicSpecularColor=[0.5 0.5 0.5 1.0]  GraphicVisPropType=SimpleVisualProperties
  Rigid Transform : sm_lib/Frames and Transforms/Rigid Transform  TranslationMethod=None  TranslationStandardOffset=0  TranslationLengthUnit=m  TranslationStandardAxis=+X  TranslationCartesianOffset=[0 0 0]  TranslationROffset=0  TranslationROffsetUnits=m  TranslationZOffset=0  TranslationZOffsetUnits=m  TranslationThetaOffset=0  TranslationThetaOffsetUnits=deg  RotationMethod=None  RotationAngleUnits=deg  RotationStandardAxis=+Z  RotationAngle=0.0  RotationArbitraryAxis=[0 0 1]  FollAlignAxisA=+X  BaseAlignAxisA=+Y  FollAlignAxisB=+Y  BaseAlignAxisB=+Z  RotationSequenceAxes=FollowerAxes  RotationSequence=XYX  RotationSequenceAngles=[0 0 0]  RotationSequenceAnglesUnits=deg  RotationMatrix=[1 0 0; 0 1 0; 0 0 1]
  Rigid Transform1 : sm_lib/Frames and Transforms/Rigid Transform  TranslationMethod=None  TranslationStandardOffset=0  TranslationLengthUnit=m  TranslationStandardAxis=-X  TranslationCartesianOffset=[0 0 0]  TranslationROffset=0  TranslationROffsetUnits=m  TranslationZOffset=0  TranslationZOffsetUnits=m  TranslationThetaOffset=0  TranslationThetaOffsetUnits=deg  RotationMethod=None  RotationAngleUnits=deg  RotationStandardAxis=-X  RotationAngle=0.0  RotationArbitraryAxis=[0 0 1]  FollAlignAxisA=+X  BaseAlignAxisA=+Y  FollAlignAxisB=+Y  BaseAlignAxisB=+Z  RotationSequenceAxes=FollowerAxes  RotationSequence=XYX  RotationSequenceAngles=[0 0 0]  RotationSequenceAnglesUnits=deg  RotationMatrix=[1 0 0; 0 1 0; 0 0 1]
  Rigid Transform2 : PMIOPort  Side=Left
  Rigid Transform3 : PMIOPort  Port=2  Side=Right
  connections:
  Rigid Transform1/LConn1 -- Rigid Transform/LConn1 -- Brick Solid/RConn1
  Rigid Transform/RConn1 -- Rigid Transform3/RConn1
  Rigid Transform2/RConn1 -- Rigid Transform1/RConn1

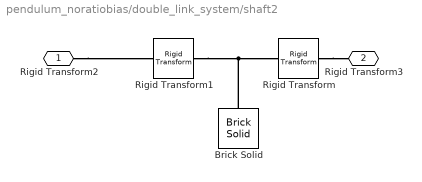
== system pendulum_noratiobias/double_link_system/shaft2 ==
  Brick Solid : sm_lib/Body Elements/Brick Solid  GraphicAmbientColor=[0.15 0.15 0.15 1.0]  BasedOnType=Density  BrickDimensions=[L W H]  BrickDimensionUnits=m  CenterOfMass=[0 0 0]  CenterOfMassUnits=m  GraphicDiffuseColor=rgb  Density=2700  DensityUnits=kg/m^3  DoExposeReferenceFrame=on  GraphicEmissiveColor=[0.0 0.0 0.0 1.0]  ExportEntireGeometry=off  SerializedFrames=<Frames/>  MarkerShape=Sphere  MarkerSize=10  GraphicType=FromGeometry  InertiaType=Custom  Mass=M  MassUnits=kg  MomentsOfInertia=[Ixx Iyy Izz]  MomentsOfInertiaUnits=kg*m^2  GraphicOpacity=1.0  ProductsOfInertia=[0 0 0]  ProductsOfInertiaUnits=kg*m^2  GraphicShininess=75  GraphicSpecularColor=[0.5 0.5 0.5 1.0]  GraphicVisPropType=SimpleVisualProperties
  Rigid Transform : sm_lib/Frames and Transforms/Rigid Transform  TranslationMethod=None  TranslationStandardOffset=0  TranslationLengthUnit=m  TranslationStandardAxis=+X  TranslationCartesianOffset=[0 0 0]  TranslationROffset=0  TranslationROffsetUnits=m  TranslationZOffset=0  TranslationZOffsetUnits=m  TranslationThetaOffset=0  TranslationThetaOffsetUnits=deg  RotationMethod=None  RotationAngleUnits=deg  RotationStandardAxis=+Z  RotationAngle=0.0  RotationArbitraryAxis=[0 0 1]  FollAlignAxisA=+X  BaseAlignAxisA=+Y  FollAlignAxisB=+Y  BaseAlignAxisB=+Z  RotationSequenceAxes=FollowerAxes  RotationSequence=XYX  RotationSequenceAngles=[0 0 0]  RotationSequenceAnglesUnits=deg  RotationMatrix=[1 0 0; 0 1 0; 0 0 1]
  Rigid Transform1 : sm_lib/Frames and Transforms/Rigid Transform  TranslationMethod=None  TranslationStandardOffset=0  TranslationLengthUnit=m  TranslationStandardAxis=-X  TranslationCartesianOffset=[0 0 0]  TranslationROffset=0  TranslationROffsetUnits=m  TranslationZOffset=0  TranslationZOffsetUnits=m  TranslationThetaOffset=0  TranslationThetaOffsetUnits=deg  RotationMethod=None  RotationAngleUnits=deg  RotationStandardAxis=-X  RotationAngle=0.0  RotationArbitraryAxis=[0 0 1]  FollAlignAxisA=+X  BaseAlignAxisA=+Y  FollAlignAxisB=+Y  BaseAlignAxisB=+Z  RotationSequenceAxes=FollowerAxes  RotationSequence=XYX  RotationSequenceAngles=[0 0 0]  RotationSequenceAnglesUnits=deg  RotationMatrix=[1 0 0; 0 1 0; 0 0 1]
  Rigid Transform2 : PMIOPort  Side=Left
  Rigid Transform3 : PMIOPort  Port=2  Side=Right
  connections:
  Rigid Transform1/LConn1 -- Rigid Transform/LConn1 -- Brick Solid/RConn1
  Rigid Transform/RConn1 -- Rigid Transform3/RConn1
  Rigid Transform2/RConn1 -- Rigid Transform1/RConn1

== matlab function pendulum_noratiobias/Subsystem4/tow2_phi_Function ==
  data: q1_vec input; q2_vec input; phi output; s2_vec input
function phi = tow2_phi(q1_vec,q2_vec,s2_vec)
q1 = q1_vec(1);
q2 = q2_vec(1);

phi2 = q1_vec(3)*cos(q2)+q2_vec(2)*q2_vec(2)*sin(q2);

phi = [q1_vec(3)+q2_vec(3);phi2;cos(q1+q2)*9.81;s2_vec(3)];

== matlab function pendulum_noratiobias/tow1_phi_Function ==
  data: s1_vec input; phi output; q1_vec input; s2_vec input; q2_vec input
function phi = tow1_phi(s1_vec,q1_vec,s2_vec,q2_vec)
s1 = s1_vec(1);
s1_d = s1_vec(2);
s1_dd = s1_vec(3);
q1 = q1_vec(1);
q1_d = q1_vec(2);
q1_dd = q1_vec(3);
s2 = s2_vec(1);
s2_d = s2_vec(2);
s2_dd = s2_vec(3);
q2 = q2_vec(1);
q2_d = q2_vec(2);
q2_dd = q2_vec(3);

phi1 = q1_dd;
phi2 = q2_dd;
phi3 = 2*cos(q2)*q1_dd + cos(q2)*d2_dd - sin(q2)*d2_d^2 - 2*sin(q2)*q1_d*q2_d;
phi4 = cos(q1+q2)*9.81;
phi5 = cos(q1)*9.81;
phi6 = s1_dd;
phi = [phi1;phi2;phi3;phi4;phi5;phi6];

== matlab function pendulum_noratiobias/Subsystem1/J1_phi_Function ==
  data: s1_vec input; phi output; q1_vec input
function phi = J2_phi(s1_vec,q1_vec)
s1 = s1_vec(1);
s1_d = s1_vec(2);
s1_dd = s1_vec(3);
q1 = q1_vec(1);
q1_d = q1_vec(2);
q1_dd = q1_vec(3);

phi1 = s1_dd;
phi2 = s1-q1;
phi3 = s1_d-q1_d;

phi = [phi1;phi2;phi3];

== matlab function pendulum_noratiobias/Subsystem2/J1_phi_Function ==
  data: s1_vec input; phi output; q1_vec input
function phi = J1_phi(s1_vec,q1_vec)
s1 = s1_vec(1);
s1_d = s1_vec(2);
s1_dd = s1_vec(3);
q1 = q1_vec(1);
q1_d = q1_vec(2);
q1_dd = q1_vec(3);

phi1 = s1_dd;
phi2 = s1-q1;
phi3 = s1_d-q1_d;

phi = [phi1;phi2;phi3];

== matlab function pendulum_noratiobias/Subsystem3/link_phi_Function ==
  data: q1_vec input; q2_vec input; phi output
function phi = J1_phi(q1_vec,q2_vec)
q1 = q1_vec(1);
q1_d = q1_vec(2);
q2 = q2_vec(1);
q2_d = q2_vec(2);

phi1 = -q1_d*sin(q1);
phi2 = -q1_d*sin(q1+q2)-q2_d*sin(q1+q2);

phi = [phi1;phi2];
